simulink model "modelo_01"  (R2022a)
settings: Solver=VariableStepAuto  StartTime=0.0  StopTime=10.0  RelTol=1e-3
settings Model: Creator=patri  LastModifiedBy=patri

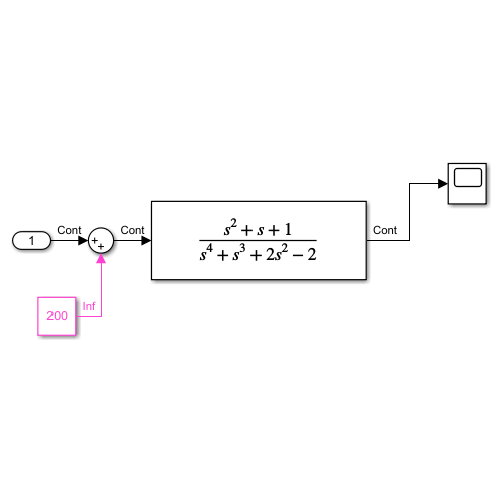
[thumbnail: Simulink's stored preview of the top-level diagram]
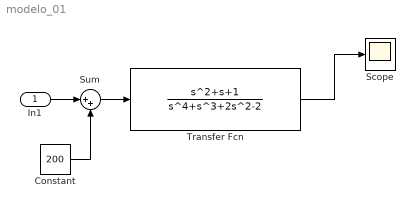
== system modelo_01 ==
  In1 : Inport
  Constant : Constant  Value=200
  Scope : Scope
  Sum : Sum  Inputs=|++
  Transfer Fcn : TransferFcn  Numerator=[1 1 1]  Denominator=[1 1 2 0 -2]
  wires:
  Sum/1 -> Transfer Fcn/1
  In1/1 -> Sum/1
  Transfer Fcn/1 -> Scope/1
  Constant/1 -> Sum/2
